simulink model "ffb_vortexdiagnostic_sweep_debug"  (Simulink 8.6)
settings: Solver=FixedStepAuto  StartTime=0.0  StopTime=dp_ts.Time(end)  FixedStep=uavsim.simConfig.tsample_model  RelTol=1e-3
model workspace (MAT data in the model file):
  VortexSig = Simulink.Signal
  VortexSig.DataType = 'Bus: VortexStates'
  VortexSig.Units = 'auto'
  VortexSig.Dimensions = [10 1]
  VortexSig.DimensionsMode = 'Fixed'
  VortexSig.Complexity = 'real'
  VortexSig.SampleTime = -1
  VortexSig.SamplingMode = 'auto'
  VortexSig.InitialValue = 'VortexStates_MATLABStruct_array'
undefined symbols (not defined in the file or in its folder): ffb_vortexdiagnostic_par, findclosemultiple, uavsim
libraries: formationFlyingBlockset x2, aerolibtransform2 x2, uavsimBlockset_UAV3DInterface x2, aerolibanimutils x1
settings Model: Creator=j.bolting  LastModifiedBy=j.bolting
settings SolverCC: AutoInsertRateTranBlk=on
settings DataIOCC: SaveFormat=Dataset  SignalLoggingSaveFormat=Dataset
settings OptimizationCC: ExpressionDepthLimit=128
settings DebuggingCC: UnderspecifiedInitializationDetection=Simplified  MergeDetectMultiDrivingBlocksExec=error  SolverPrmCheckMsg=none  FcnCallInpInsideContextMsg=EnableAllAsError  StateNameClashWarn=none
settings HardwareCC: ProdBitPerPointer=64  ProdLargestAtomicFloat=Float  ProdIntDivRoundTo=Zero  ProdEndianess=LittleEndian  ProdWordSize=64  ProdHWDeviceType=Intel->x86-64 (Windows64)
settings GRTTargetCC: GeneratePreprocessorConditionals=Use local settings  CombineOutputUpdateFcns=on  GRTInterface=off
settings ConfigComp: CovModelRefEnable=off

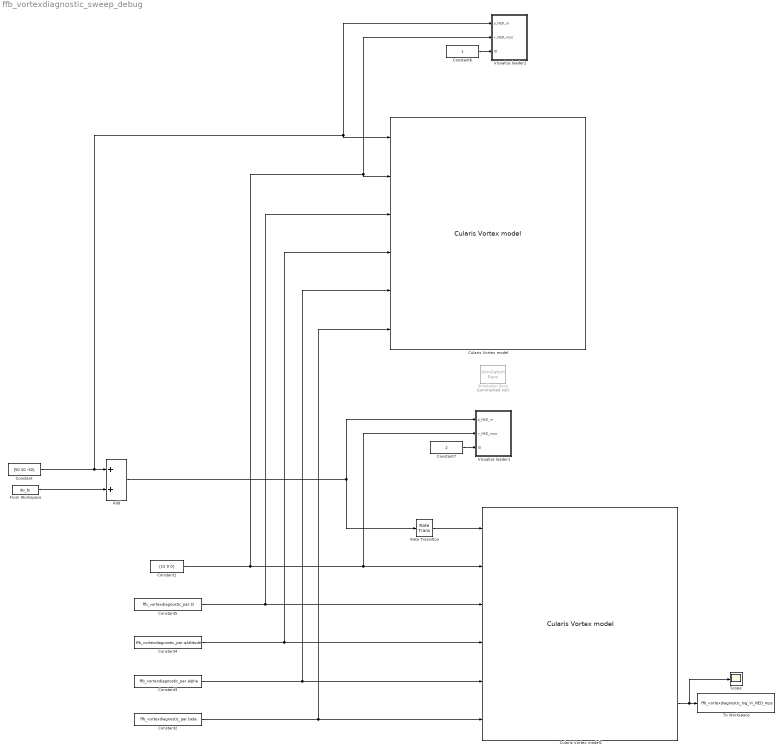
== system ffb_vortexdiagnostic_sweep_debug ==
  Add : Sum
  Constant : Constant  Value=[50 50 -50]
  Constant1 : Constant  Value=[15 0 0]
  Constant2 : Constant  Value=ffb_vortexdiagnostic_par.beta
  Constant3 : Constant  Value=ffb_vortexdiagnostic_par.alpha
  Constant4 : Constant  Value=ffb_vortexdiagnostic_par.qAttitude
  Constant5 : Constant  Value=ffb_vortexdiagnostic_par.Cl
  Constant6 : Constant
  Constant7 : Constant  Value=2
  Cularis Vortex model : formationFlyingBlockset/Cularis Vortex model  mask_ID=1
  Cularis Vortex model1 : formationFlyingBlockset/Cularis Vortex model  mask_ID=2
  From Workspace : FromWorkspace  VariableName=dp_ts  SampleTime=uavsim.simConfig.tsample_model
  Rate Transition : RateTransition
  Scope : Scope
  Simulation Pace : aerolibanimutils/Simulation Pace  Commented=on  SimulationPace=0.1  SleepMode=MATLAB Thread  OutputPaceError=off  SampleTime=findclosemultiple(1/30, uavsim.simConfig.tsample_model)
  To Workspace : ToWorkspace  VariableName=ffb_vortexdiagnostic_log_Vi_NED_mps  SaveFormat=Timeseries  SampleTime=-1
  Visualize leader1 : Subsystem  AncestorBlock=formationFlyingBlockset/Visualize leader  TreatAsAtomicUnit=on  SystemSampleTime=uavsim.simConfig.tsample_UAV3D  mask{mask_3dmodel=1}
      mask prompts: mask_3dmodel "3D model"
      mask TypeOptions mask_3dmodel: 0 | 1 | 2 | 3
  Visualize leader2 : Subsystem  AncestorBlock=formationFlyingBlockset/Visualize leader  TreatAsAtomicUnit=on  SystemSampleTime=uavsim.simConfig.tsample_UAV3D  mask{mask_3dmodel=1}
      mask prompts: mask_3dmodel "3D model"
      mask TypeOptions mask_3dmodel: 0 | 1 | 2 | 3
  wires:
  Constant7/1 -> Visualize leader1/3(ID)
  Cularis Vortex model1/3 -> Scope/1, To Workspace/1
  Constant5/1 -> Cularis Vortex model/3, Cularis Vortex model1/3
  Constant4/1 -> Cularis Vortex model/4, Cularis Vortex model1/4
  Constant3/1 -> Cularis Vortex model/5, Cularis Vortex model1/5
  Add/1 -> Visualize leader1/1(p_NED_m), Rate Transition/1
  Constant2/1 -> Cularis Vortex model/6, Cularis Vortex model1/6
  Constant6/1 -> Visualize leader2/3(ID)
  Constant1/1 -> Visualize leader2/2(v_NED_mps), Cularis Vortex model/2, Visualize leader1/2(v_NED_mps), Cularis Vortex model1/2
  Constant/1 -> Visualize leader2/1(p_NED_m), Cularis Vortex model/1, Add/1
  From Workspace/1 -> Add/2
  Rate Transition/1 -> Cularis Vortex model1/1

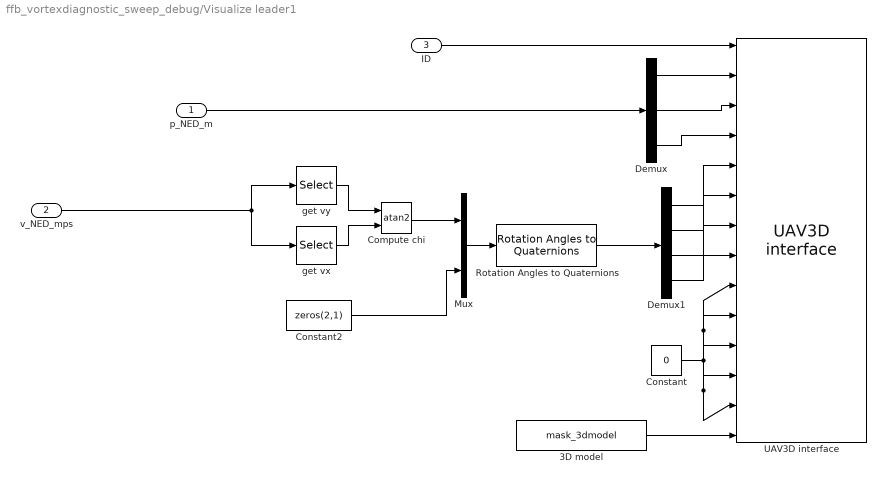
== system ffb_vortexdiagnostic_sweep_debug/Visualize leader1 ==
  p_NED_m : Inport
  v_NED_mps : Inport  Port=2
  ID : Inport  Port=3
  3D model : Constant  Value=mask_3dmodel
  Compute chi : Trigonometry  Operator=atan2
  Constant : Constant  Value=0
  Constant2 : Constant  Value=zeros(2,1)
  Demux : Demux  Outputs=3
  Demux1 : Demux
  Mux : Mux  Inputs=2
  Rotation Angles to Quaternions : aerolibtransform2/Rotation Angles to Quaternions  rotationOrder=ZYX
  UAV3D interface : uavsimBlockset_UAV3DInterface/UAV3D interface  ip='localhost'  udpport=4445
  get vx : Selector  InputPortWidth=3  IndexOptions=Index vector (dialog)  Indices=1  OutputSizes=1
  get vy : Selector  InputPortWidth=3  IndexOptions=Index vector (dialog)  Indices=2  OutputSizes=1
  wires:
  Demux/1 -> UAV3D interface/2
  Demux/2 -> UAV3D interface/3
  Demux/3 -> UAV3D interface/4
  Demux1/1 -> UAV3D interface/5
  Demux1/2 -> UAV3D interface/6
  Demux1/4 -> UAV3D interface/8
  get vy/1 -> Compute chi/1
  get vx/1 -> Compute chi/2
  Constant2/1 -> Mux/2
  Mux/1 -> Rotation Angles to Quaternions/1
  Rotation Angles to Quaternions/1 -> Demux1/1
  Compute chi/1 -> Mux/1
  Demux1/3 -> UAV3D interface/7
  Constant/1 -> UAV3D interface/13, UAV3D interface/12, UAV3D interface/11, UAV3D interface/10, UAV3D interface/9
  3D model/1 -> UAV3D interface/14
  ID/1 -> UAV3D interface/1
  p_NED_m/1 -> Demux/1
  v_NED_mps/1 -> get vy/1, get vx/1

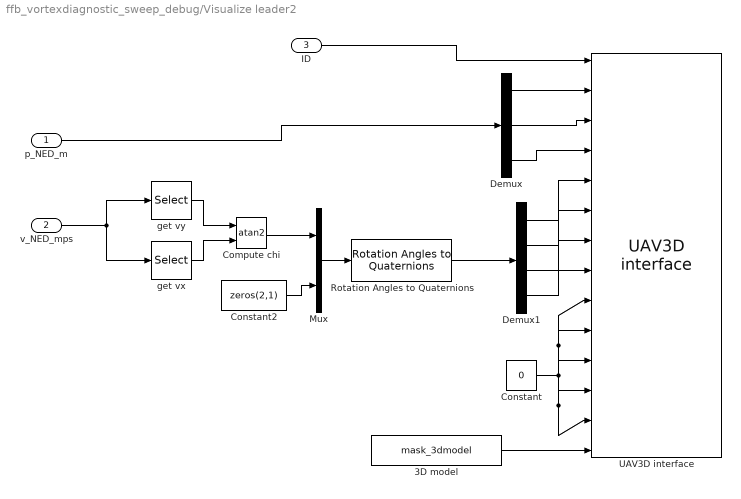
== system ffb_vortexdiagnostic_sweep_debug/Visualize leader2 ==
  p_NED_m : Inport
  v_NED_mps : Inport  Port=2
  ID : Inport  Port=3
  3D model : Constant  Value=mask_3dmodel
  Compute chi : Trigonometry  Operator=atan2
  Constant : Constant  Value=0
  Constant2 : Constant  Value=zeros(2,1)
  Demux : Demux  Outputs=3
  Demux1 : Demux
  Mux : Mux  Inputs=2
  Rotation Angles to Quaternions : aerolibtransform2/Rotation Angles to Quaternions  rotationOrder=ZYX
  UAV3D interface : uavsimBlockset_UAV3DInterface/UAV3D interface  ip='localhost'  udpport=4445
  get vx : Selector  InputPortWidth=3  IndexOptions=Index vector (dialog)  Indices=1  OutputSizes=1
  get vy : Selector  InputPortWidth=3  IndexOptions=Index vector (dialog)  Indices=2  OutputSizes=1
  wires:
  3D model/1 -> UAV3D interface/14
  ID/1 -> UAV3D interface/1
  Constant/1 -> UAV3D interface/9, UAV3D interface/10, UAV3D interface/11, UAV3D interface/12, UAV3D interface/13
  Demux1/3 -> UAV3D interface/7
  Compute chi/1 -> Mux/1
  Rotation Angles to Quaternions/1 -> Demux1/1
  Mux/1 -> Rotation Angles to Quaternions/1
  Constant2/1 -> Mux/2
  v_NED_mps/1 -> get vx/1, get vy/1
  get vx/1 -> Compute chi/2
  get vy/1 -> Compute chi/1
  p_NED_m/1 -> Demux/1
  Demux1/4 -> UAV3D interface/8
  Demux1/2 -> UAV3D interface/6
  Demux1/1 -> UAV3D interface/5
  Demux/3 -> UAV3D interface/4
  Demux/2 -> UAV3D interface/3
  Demux/1 -> UAV3D interface/2
